simulink model "Runge-Kutta odometry localization"  (R2020a)
settings: Solver=VariableStepAuto  StartTime=0.0  StopTime=10.0  RelTol=1e-3
InitFcn:
  | T_s=0.01
settings Model: Creator=ThinkPad  LastModifiedBy=ThinkPad

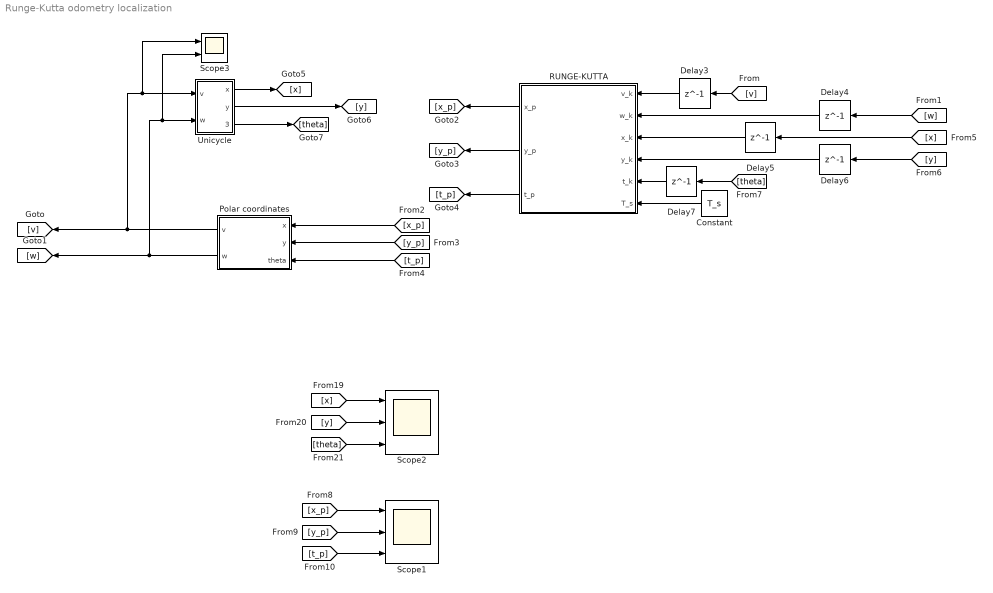
== system Runge-Kutta odometry localization ==
  Constant : Constant  Value=T_s
  Delay3 : Delay  DelayLength=1  InitialCondition=0  SampleTime=T_s
  Delay4 : Delay  DelayLength=1  InitialCondition=0  SampleTime=T_s
  Delay5 : Delay  DelayLength=1  InitialCondition=5  SampleTime=T_s
  Delay6 : Delay  DelayLength=1  InitialCondition=2  SampleTime=T_s
  Delay7 : Delay  DelayLength=1  InitialCondition=pi/2  SampleTime=T_s
  Polar coordinates : MATLAB Function  TreatAsAtomicUnit=on
  RUNGE-KUTTA : MATLAB Function  TreatAsAtomicUnit=on  SystemSampleTime=T_s
  Scope1 : Scope  NumInputPorts=3
  Scope2 : Scope  NumInputPorts=3
  Scope3 : Scope  NumInputPorts=2
  Unicycle : Subsystem
  wires:
  Polar coordinates/2(w) -> Scope3/2, Unicycle/2(w), [w]
  Unicycle/2(y) -> [y]
  Polar coordinates/1(v) -> Scope3/1, Unicycle/1(v), [v]
  [theta] -> Delay7/1
  Unicycle/3(theta) -> [theta]
  RUNGE-KUTTA/3(t_p) -> [t_p]
  Unicycle/1(x) -> [x]
  Constant/1 -> RUNGE-KUTTA/6(T_s)
  [y_p] -> Polar coordinates/2(y)
  [w] -> Delay4/1
  RUNGE-KUTTA/2(y_p) -> [y_p]
  [x] -> Delay5/1
  [t_p] -> Polar coordinates/3(theta)
  RUNGE-KUTTA/1(x_p) -> [x_p]
  [y] -> Delay6/1
  [v] -> Delay3/1
  [x_p] -> Polar coordinates/1(x)
  Delay3/1 -> RUNGE-KUTTA/1(v_k)
  Delay4/1 -> RUNGE-KUTTA/2(w_k)
  Delay5/1 -> RUNGE-KUTTA/3(x_k)
  Delay6/1 -> RUNGE-KUTTA/4(y_k)
  Delay7/1 -> RUNGE-KUTTA/5(t_k)
  [x] -> Scope2/1
  [y] -> Scope2/2
  [theta] -> Scope2/3
  [x_p] -> Scope1/1
  [y_p] -> Scope1/2
  [t_p] -> Scope1/3

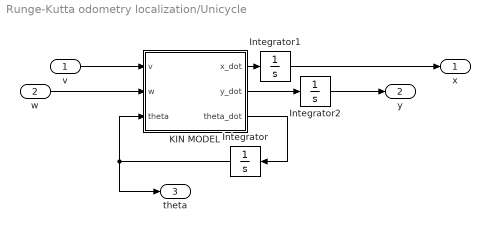
== system Runge-Kutta odometry localization/Unicycle ==
  v : Inport
  w : Inport  Port=2
  Integrator : Integrator  InitialCondition=pi/2
  Integrator1 : Integrator  InitialCondition=5
  Integrator2 : Integrator  InitialCondition=2
  KIN MODEL : MATLAB Function  TreatAsAtomicUnit=on
  x : Outport
  y : Outport  Port=2
  theta : Outport  Port=3
  wires:
  KIN MODEL/3(theta_dot) -> Integrator/1
  v/1 -> KIN MODEL/1(v)
  KIN MODEL/2(y_dot) -> Integrator2/1
  Integrator/1 -> theta/1, KIN MODEL/3(theta)
  Integrator2/1 -> y/1
  KIN MODEL/1(x_dot) -> Integrator1/1
  w/1 -> KIN MODEL/2(w)
  Integrator1/1 -> x/1

== matlab function Runge-Kutta odometry localization/Unicycle/KIN MODEL ==
  data: v input; x_dot output; w input; y_dot output; theta_dot output; theta input
function [x_dot,y_dot,theta_dot] = fcn(v,w,theta)
x_dot=cos(theta)*v
y_dot=sin(theta)*v
theta_dot=w;

== matlab function Runge-Kutta odometry localization/RUNGE-KUTTA ==
  data: v_k input; x_p output; w_k input; x_k input; y_k input; t_k input; y_p output; t_p output; T_s input
function [x_p,y_p,t_p] = fcn(v_k,w_k,x_k,y_k,t_k,T_s)

x_p=x_k+v_k*T_s*cos(t_k+0.5*w_k*T_s);
y_p=y_k+v_k*T_s*sin(t_k+0.5*w_k*T_s);
t_p=t_k+w_k*T_s;

== matlab function Runge-Kutta odometry localization/Polar coordinates ==
  data: x input; v output; y input; theta input; w output
function [v,w] = fcn(x,y,theta)
rho=sqrt(x^2+y^2);
gamma=atan2(y,x)-theta+pi;
delta=gamma+theta;

k_1=2;
k_2=7;
k_3=1;
v=k_1*rho*cos(gamma);
w=k_2*gamma+k_1*sin(gamma)*cos(gamma)*(1+k_3*delta/gamma);
